simulink model "comb_d"  (Simulink 5.0)
settings: Solver=ode23s  StartTime=t0  StopTime=tf  RelTol=1e-8  AbsTol=1.0e-8
values from neighbouring files (symbols this model uses):
  A = [1 -0.43]    [ibm_pp.m]    (also in unstb.m = [1 2 -8])
  B = 0.47    [ibm_pp.m]    (also in unstb.m = [1 -3])
  Delta = [1 -1]    [ibm_pp.m]    (also in motor_pd.m = 1)
  st = 1    [ant-old.m]    (also in ibm_pp.m; motor_pd.m; unstb.m)
  Ts = 0.01; [B,A,k] = myc2d(G,Ts)    [ant-old.m]    (also in ibm_pp.m = 1; motor_pd.m = 0.25; [B,A,k] = myc2d(G,Ts); unstb.m = 1)
undefined symbols (not defined in the file or in its folder): R, S, TM, zk
settings Model: Creator=kannanm  LastModifiedBy=kannan  ExtModeAutoUpdateStatusClock=off

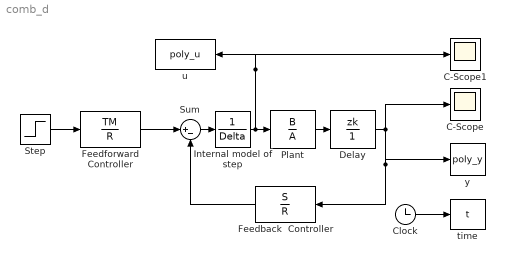
== system comb_d ==
  C-Scope : Scope
      settings: YMin=-5e+14  YMax=8.5e+15
  C-Scope1 : Scope
      settings: YMin=0  YMax=1.2
  Clock : Clock
      settings: Decimation=10
  Delay : DiscreteFilter  Numerator=zk  Denominator=1  SampleTime=Ts
  Feedback  Controller : DiscreteFilter  Orientation=left  Numerator=S  Denominator=R  SampleTime=Ts
  Feedforward Controller : DiscreteFilter  Numerator=TM  Denominator=R  SampleTime=Ts
  Internal model of step : DiscreteFilter  Numerator=1  Denominator=Delta  SampleTime=Ts
  Plant : DiscreteFilter  Numerator=B  Denominator=A  SampleTime=Ts
  Step : Step  Time=0  After=st  SampleTime=Ts
  Sum : Sum  Inputs=|+-  SaturateOnIntegerOverflow=on
  time : ToWorkspace  VariableName=t  SampleTime=Ts  SaveFormat=Array
  u : ToWorkspace  VariableName=poly_u  SampleTime=Ts  SaveFormat=Array
  y : ToWorkspace  VariableName=poly_y  SampleTime=Ts  SaveFormat=Array
  wires:
  Step/1 -> Feedforward Controller/1
  Feedforward Controller/1 -> Sum/1
  Feedback  Controller/1 -> Sum/2
  Clock/1 -> time/1
  Delay/1 -> Feedback  Controller/1, y/1, C-Scope/1
  Plant/1 -> Delay/1
  Sum/1 -> Internal model of step/1
  Internal model of step/1 -> Plant/1, u/1, C-Scope1/1
